simulink model "Problem_4"  (R2020a)
settings: Solver=VariableStepAuto  StartTime=0.0  StopTime=10.0  RelTol=1e-3
undefined symbols (not defined in the file or in its folder): b, J, Kd, Ke, Ki, Kp, Kt, L, R
settings Model: Creator=Saqlain  LastModifiedBy=Saqlain

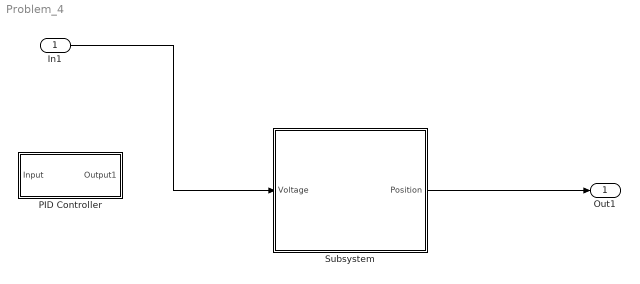
== system Problem_4 ==
  In1 : Inport
  PID Controller : Subsystem
  Subsystem : Subsystem
  Out1 : Outport
  wires:
  In1/1 -> Subsystem/1(Voltage)
  Subsystem/1(Position) -> Out1/1

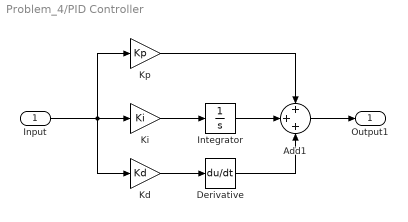
== system Problem_4/PID Controller ==
  Input : Inport
  Add1 : Sum  Inputs=+++
  Derivative : Derivative
  Integrator : Integrator
  Kd : Gain  Gain=Kd
  Ki : Gain  Gain=Ki
  Kp : Gain  Gain=Kp
  Output1 : Outport  OutDataTypeStr=double  PortDimensions=1  SampleTime=0
  wires:
  Integrator/1 -> Add1/2
  Kp/1 -> Add1/1
  Ki/1 -> Integrator/1
  Input/1 -> Kp/1, Kd/1, Ki/1
  Add1/1 -> Output1/1
  Derivative/1 -> Add1/3
  Kd/1 -> Derivative/1

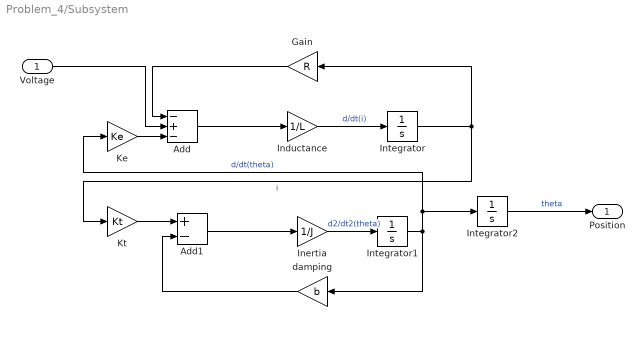
== system Problem_4/Subsystem ==
  Voltage : Inport
  Add : Sum  Inputs=-+-
  Add1 : Sum  Inputs=+-
  Gain : Gain  Gain=R
  Inductance : Gain  Gain=1/L
  Inertia : Gain  Gain=1/J
  Integrator : Integrator
  Integrator1 : Integrator
  Integrator2 : Integrator
  Ke : Gain  Gain=Ke
  Kt : Gain  Gain=Kt
  damping : Gain  Gain=b
  Position : Outport
  wires:
  Add1/1 -> Inertia/1
  Add/1 -> Inductance/1
  Integrator1/1 -> Ke/1, Integrator2/1, damping/1  "d/dt(theta)"
  Integrator/1 -> Gain/1, Kt/1  "i"
  Inertia/1 -> Integrator1/1  "d2/dt2(theta)"
  Inductance/1 -> Integrator/1  "d/dt(i)"
  Kt/1 -> Add1/1
  Voltage/1 -> Add/2
  damping/1 -> Add1/2
  Ke/1 -> Add/3
  Gain/1 -> Add/1
  Integrator2/1 -> Position/1  "theta"
